simulink model "Sub4"  (R2024a)
settings: Solver=FixedStepDiscrete  StartTime=0.0  StopTime=4.5  FixedStep=75e-6  RelTol=1e-3  EnableMultiTasking=on
undefined symbols (not defined in the file or in its folder): D1, D11, Delta
libraries: spsSeriesRLCBranchLib x41, spsLoadFlowBusLib x29, spsDistributedParametersLineLib x19, spsThreePhaseSeriesRLCLoadLib x15, spsThreePhaseTransformerTwoWindingsLib x13, spsThreePhaseParallelRLCLoadLib x11, spsThreePhaseVIMeasurementLib x11, spsSynchronousMachinepuStandardLib x7, spsExcitationSystemLib x7, spsHydraulicTurbineandGovernorLib x7, spsGenericPowerSystemStabilizerLib x7, spsMultiBandPowerSystemStabilizerLib x7
(part 2 of 5)

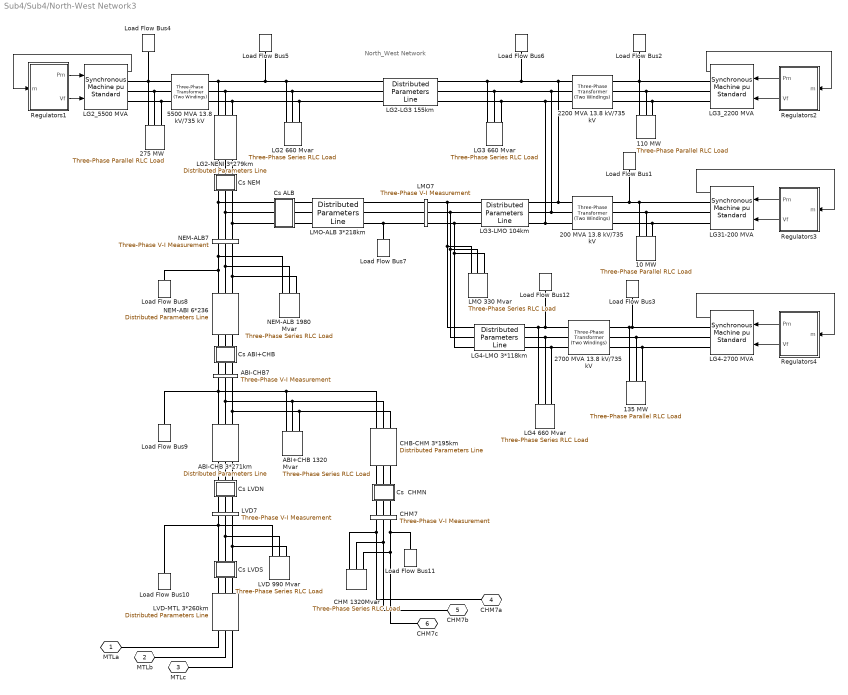
== system Sub4/Sub4/North-West Network3 ==
  note: North_West Network
  10 MW : spsThreePhaseParallelRLCLoadLib/Three-Phase Parallel RLC Load  LConnTagsString=A|B|C  Configuration=Y (grounded)  NominalVoltage=(13800)*1  Vabc=[1e3 1e3 1e3]  Vabcp=[1e3 1e3 1e3]  NominalFrequency=60  UnbalancedPower=off  ActivePower=10000000  InductivePower=0  CapacitivePower=0  Pabc=[10e3 9e3 11e3]  QLabc=[100 90 110]  QCabc=[100 90 110]  Pabcp=[10e3 9e3 11e3]  QLabcp=[100 90 110]  QCabcp=[100 90 110]  Measurements=None  LoadType=constant PQ
  110 MW : spsThreePhaseParallelRLCLoadLib/Three-Phase Parallel RLC Load  LConnTagsString=A|B|C  Configuration=Y (grounded)  NominalVoltage=(13800)*1  Vabc=[1e3 1e3 1e3]  Vabcp=[1e3 1e3 1e3]  NominalFrequency=60  UnbalancedPower=off  ActivePower=110000000  InductivePower=0  CapacitivePower=0  Pabc=[10e3 9e3 11e3]  QLabc=[100 90 110]  QCabc=[100 90 110]  Pabcp=[10e3 9e3 11e3]  QLabcp=[100 90 110]  QCabcp=[100 90 110]  Measurements=None  LoadType=constant PQ
  135 MW : spsThreePhaseParallelRLCLoadLib/Three-Phase Parallel RLC Load  LConnTagsString=A|B|C  Configuration=Y (grounded)  NominalVoltage=(13800)*1  Vabc=[1e3 1e3 1e3]  Vabcp=[1e3 1e3 1e3]  NominalFrequency=60  UnbalancedPower=off  ActivePower=135000000  InductivePower=0  CapacitivePower=0  Pabc=[10e3 9e3 11e3]  QLabc=[100 90 110]  QCabc=[100 90 110]  Pabcp=[10e3 9e3 11e3]  QLabcp=[100 90 110]  QCabcp=[100 90 110]  Measurements=None  LoadType=constant PQ
  200 MVA 13.8 kV/735 kV : spsThreePhaseTransformerTwoWindingsLib/Three-Phase Transformer (Two Windings)  Winding1Connection=Delta (D1)  Winding2Connection=Yg  CoreType=Three single-phase transformers  SetSaturation=off  Hysteresis=off  DataFile='basic_model'  SetInitialFlux=off  Measurements=None  UNITS=pu  NominalPower=[ 200e6 60 ]  Winding1="[ 13.8e3 0.002  0.0]"  Winding2=[ 735e3 0.002 0.12]  Rm=500  Lm=500  L0=0.5  Saturation="[ 0,0  ;  0.005,1.2  ;  1.0,1.4 ]"  InitialFluxes=[ 0.8 , -0.8 , 0.7 ]  BreakLoop=off  DiscreteSolver=Trapezoidal iterative  DataType=off  TransfoNumber=0
  2200 MVA 13.8 kV/735 kV : spsThreePhaseTransformerTwoWindingsLib/Three-Phase Transformer (Two Windings)  Winding1Connection=Delta (D1)  Winding2Connection=Yg  CoreType=Three single-phase transformers  SetSaturation=off  Hysteresis=off  DataFile='basic_model'  SetInitialFlux=off  Measurements=None  UNITS=pu  NominalPower=[ 2200e6 60 ]  Winding1="[ 13.8e3 0.002  0.0]"  Winding2=[ 735e3 0.002 0.12]  Rm=500  Lm=500  L0=0.5  Saturation="[ 0,0  ;  0.005,1.2  ;  1.0,1.4 ]"  InitialFluxes=[ 0.8 , -0.8 , 0.7 ]  BreakLoop=off  DiscreteSolver=Trapezoidal iterative  DataType=off  TransfoNumber=0
  2700 MVA 13.8 kV/735 kV : spsThreePhaseTransformerTwoWindingsLib/Three-Phase Transformer (Two Windings)  Winding1Connection=Delta (D1)  Winding2Connection=Yg  CoreType=Three single-phase transformers  SetSaturation=off  Hysteresis=off  DataFile='basic_model'  SetInitialFlux=off  Measurements=None  UNITS=pu  NominalPower=[ 2700e6 60 ]  Winding1="[ 13.8e3 0.002  0.0]"  Winding2=[ 735e3 0.002 0.12]  Rm=500  Lm=500  L0=0.5  Saturation="[ 0,0  ;  0.005,1.2  ;  1.0,1.4 ]"  InitialFluxes=[ 0.8 , -0.8 , 0.7 ]  BreakLoop=off  DiscreteSolver=Trapezoidal iterative  DataType=off  TransfoNumber=0
  275 MW : spsThreePhaseParallelRLCLoadLib/Three-Phase Parallel RLC Load  LConnTagsString=A|B|C  Configuration=Y (grounded)  NominalVoltage=(13800)*1  Vabc=[1e3 1e3 1e3]  Vabcp=[1e3 1e3 1e3]  NominalFrequency=60  UnbalancedPower=off  ActivePower=275000000  InductivePower=0  CapacitivePower=0  Pabc=[10e3 9e3 11e3]  QLabc=[100 90 110]  QCabc=[100 90 110]  Pabcp=[10e3 9e3 11e3]  QLabcp=[100 90 110]  QCabcp=[100 90 110]  Measurements=None  LoadType=constant PQ
  5500 MVA 13.8 kV/735 kV : spsThreePhaseTransformerTwoWindingsLib/Three-Phase Transformer (Two Windings)  Winding1Connection=Delta (D1)  Winding2Connection=Yg  CoreType=Three single-phase transformers  SetSaturation=off  Hysteresis=off  DataFile='basic_model'  SetInitialFlux=off  Measurements=None  UNITS=pu  NominalPower=[ 5500e6 60 ]  Winding1="[ 13.8e3 0.002  0.0]"  Winding2=[ 735e3 0.002 0.12]  Rm=500  Lm=500  L0=0.5  Saturation="[ 0,0  ;  0.005,1.2  ;  1.0,1.4 ]"  InitialFluxes=[ 0.8 , -0.8 , 0.7 ]  BreakLoop=off  DiscreteSolver=Trapezoidal iterative  DataType=off  TransfoNumber=0
  ABI+CHB 1320 Mvar : spsThreePhaseSeriesRLCLoadLib/Three-Phase Series RLC Load  LConnTagsString=A|B|C  Configuration=Y (grounded)  NominalVoltage=735e3  Vabc=[1e3 1e3 1e3]  Vabcp=[1e3 1e3 1e3]  NominalFrequency=60  UnbalancedPower=off  ActivePower=4400000  InductivePower=1320e6  CapacitivePower=0  Pabc=[10e3 9e3 11e3]  QLabc=[100 90 110]  QCabc=[100 90 110]  Pabcp=[10e3 9e3 11e3]  QLabcp=[100 90 110]  QCabcp=[100 90 110]  Measurements=None  LoadType=constant Z
  ABI-CHB 3*271km : spsDistributedParametersLineLib/Distributed Parameters Line  Phases=3  Length=271  Frequency=60  Resistance="[0.01273  0.3864]/3"  Inductance="[0.9337e-3  4.1264e-3]/3"  Capacitance=[12.74e-9 7.751e-9]*3  x1=[-0.001575 2.80962252870906e-08 -103484.456536303 -819305.847115616;-0.0015 2.82171345098539e-08 -80280.8596539916 -821903.919579672;-0.001425 2.83154873870267e-08 -57013.0874808114 -823844.974625968;-0.00135 2.83912052968237e-08 -33699.7399178284 -825127.4606048;-0.001275 2.84442277115065e-08 -10359.4532983786 -825750.352316497;-0.0012 2.8474512245768e-08 12989.1145095332 -825713.151830956;-0.001125 2.84820346906148e-08 36327.2990180461 -825015.888885677;-0.00105 2.84667890327198e-08 59636.4440395503 -823659.120861989;-0.000975 2.84287874592284e-08 82897.9166001574 -821643.93233949;-0.0009 2.83680603480172e-08 106093.121834615 -818971.934229054;-0.000825 2.82846562434096e-08 129203.517850757 -815645.262485085;-0.00075 2.81786418173708e-08 152210.63055161 -811666.576398077;-0.000675 2.80501018162109e-08 175096.0684033 -807039.056468812;-0.0006 2.78991389928401e-08 197841.537136968 -801766.401865916;-0.000525 2.77258740246295e-08 220428.854372927 -795852.827468807;-0.00045 2.75304454169437e-08 242839.964155374 -789303.060498376;-0.000375 2.73130093924216e-08 265056.951386051 -782122.336738124;-0.0003 2.70737397660942e-08 287062.056145297 -774316.396348756;-0.000225 2.68128278064399e-08 308837.687889058 -765891.479279586;-0.00015 2.65304820824872e-08 330366.439510495 -756854.320280412;-7.5e-05 2.62269282970877e-08 351631.101254964 -747212.143517865]  x2=[-0.001575 6.39240813487654e-08 -329701.15801167 -748762.187115756;-0.0015 6.41301801382965e-08 -308401.441010082 -757783.743021244;-0.001425 6.42850142430497e-08 -286855.19261525 -766199.538197041;-0.00135 6.43884598910107e-08 -265079.636568473 -774002.845185249;-0.001275 6.44404343893114e-08 -243092.179916078 -781187.426141657;-0.0012 6.44408961903329e-08 -220910.399094493 -787747.537822176;-0.001125 6.43898449249186e-08 -198552.025879915 -793677.936173901;-0.00105 6.4287321402669e-08 -176034.933213796 -798973.880527129;-0.000975 6.41334075793192e-08 -153377.12091549 -803631.137384973;-0.0009 6.39282264912245e-08 -130596.701293474 -807645.98380756;-0.000825 6.36719421570073e-08 -107711.88466664 -811015.21038809;-0.00075 6.33647594464432e-08 -84740.9648072501 -813736.123818384;-0.000675 6.3006923916691e-08 -61702.3043171739 -815806.549041878;-0.0006 6.2598721615998e-08 -38614.3199491035 -817224.830992327;-0.000525 6.21404788550378e-08 -15495.4678844847 -817989.83591684;-0.00045 6.1632561946062e-08 7635.77102007237 -818100.952282185;-0.000375 6.10753769100764e-08 30760.9060061072 -817558.09126364;-0.0003 6.04693691522735e-08 53861.4511945383 -816361.686815997;-0.000225 5.98150231059826e-08 76918.9403629924 -814512.695326666;-0.00015 5.91128618454214e-08 99914.9417074196 -812012.594851153;-7.5e-05 5.8363446667558e-08 122831.072576196 -808863.383931525]  x3=[-0.001575 1.30051771042059e-10 -747.841433918899 -1501.46113433961;-0.0015 1.38144212565734e-10 -705.095036949488 -1522.00231179776;-0.001425 1.46126223719561e-10 -661.784997795856 -1541.32682389527;-0.00135 1.53991423805954e-10 -617.945937840636 -1559.41922291284;-0.001275 1.61733525504303e-10 -573.612901357596 -1576.26504606354;-0.0012 1.69346339896971e-10 -528.821327497782 -1591.85082705408;-0.001125 1.7682378141661e-10 -483.607021960005 -1606.1641068496;-0.00105 1.8415987271088e-10 -438.006128368308 -1619.19344363325;-0.000975 1.91348749420646e-10 -392.055099379312 -1630.92842195254;-0.0009 1.98384664867858e-10 -345.790667542516 -1641.35966104537;-0.000825 2.05261994649362e-10 -299.249815936862 -1650.4788223388;-0.00075 2.11975241132958e-10 -252.469748607023 -1658.27861611483;-0.000675 2.18519037852121e-10 -205.487860823064 -1664.75280733764;-0.0006 2.24888153795879e-10 -158.341709187234 -1669.89622063785;-0.000525 2.31077497590397e-10 -111.068981611788 -1673.70474444954;-0.00045 2.37082121568946e-10 -63.7074671918543 -1676.17533429707;-0.000375 2.4289722572699e-10 -16.2950259974044 -1677.3060152287;-0.0003 2.4851816155924e-10 31.1304411915056 -1677.0958833954;-0.000225 2.53940435775595e-10 78.5310231820388 -1675.54510677334;-0.00015 2.5915971389301e-10 125.868828674205 -1672.65492502962;-7.5e-05 2.64171823700416e-10 173.106016550587 -1668.42764853132]  x4=[-0.001575 1.94160017785796e-10 -7080.29438162629 -14859.1258761648;-0.0015 1.90056959794632e-10 -6657.38891400296 -15053.3510061753;-0.001425 1.85801973177776e-10 -6229.16163154324 -15235.5427177154;-0.00135 1.81398459306428e-10 -5795.95485258464 -15405.5553695186;-0.001275 1.768499382822e-10 -5358.11487599796 -15563.2530560724;-0.0012 1.72160046123204e-10 -4915.99170436132 -15708.5097162588;-0.001125 1.67332531857473e-10 -4469.9387641734 -15841.2092341263;-0.00105 1.6237125452605e-10 -4020.31262332977 -15961.2455317107;-0.000975 1.57280180098122e-10 -3567.47270608789 -16068.5226538323;-0.0009 1.52063378300691e-10 -3111.78100574892 -16162.9548448011;-0.000825 1.46725019365294e-10 -2653.60179528581 -16244.4666169684;-0.00075 1.41269370694385e-10 -2193.30133614901 -16312.9928110708;-0.000675 1.35700793450036e-10 -1731.24758548273 -16368.4786483172;-0.0006 1.30023739067695e-10 -1267.80990198559 -16410.8797741782;-0.000525 1.24242745697774e-10 -803.35875065095 -16440.1622938426;-0.00045 1.18362434577919e-10 -338.265406622837 -16456.3027993123;-0.000375 1.12387506338869e-10 127.098341595695 -16459.2883881141;-0.0003 1.06322737246837e-10 592.360489344626 -16449.1166736139;-0.000225 1.00172975385444e-10 1057.14911318179 -16425.7957869249;-0.00015 9.39431367802247e-11 1521.09266819281 -16389.3443704068;-7.5e-05 8.76382014688418e-11 1983.82028499837 -16339.7915627644]  x5=0.00153261764655846  V1=ones(3,3)  V2=ones(3,3)  I1=ones(3,3)  I2=ones(3,3)  nHarmo=1  Measurements=None  Decoupling=on  VsMag0=[674275.598206343 674275.04688363 674275.387112461]  VrMag0=[668005.988427244 668005.867389034 668005.726368297]  VsAngle0=[-3.17875639507245 -123.178750059774 116.821287344148]  VrAngle0=[-19.7452308032692 -139.745250763834 100.254768207195]  IsMag0=[1378.35069563154 1378.34088888526 1378.33344706121]  IrMag0=[13525.2461163755 13525.2482026067 13525.2572474119]  IsAngle0=[-22.4561903612897 -142.456782921022 97.5438663998778]  IrAngle0=[-21.4575985540855 -141.457549208479 98.5424184650439]
      settings: AttributesFormatString=\n  LibrarySourceBlock=sps_lib/Power Grid Elements/Distributed Parameters Line
  ABI-CHB7 : spsThreePhaseVIMeasurementLib/Three-Phase V-I Measurement  VoltageMeasurement=no  SetLabelV=on  LabelV=Vabc_ABI7  Vpu=on  VpuLL=off  CurrentMeasurement=no  SetLabelI=off  LabelI=A1  Ipu=off  Pbase=100e6  Vbase=500e3  OutputType=Magnitude  PhasorSimulation=off  PSBequivalent=0
  CHB-CHM 3*195km : spsDistributedParametersLineLib/Distributed Parameters Line  Phases=3  Length=195  Frequency=60  Resistance="[0.01273  0.3864]/3"  Inductance="[0.9337e-3  4.1264e-3]/3"  Capacitance=[12.74e-9 7.751e-9]*3  x1=[-0.001125 2.84820346906148e-08 0 0;-0.00105 2.84667890327198e-08 0 0;-0.000975 2.84287874592284e-08 0 0;-0.0009 2.83680603480172e-08 0 0;-0.000825 2.82846562434096e-08 0 0;-0.00075 2.81786418173708e-08 0 0;-0.000675 2.80501018162109e-08 175096.0684033 -807039.056468812;-0.0006 2.78991389928401e-08 197841.537136968 -801766.401865916;-0.000525 2.77258740246295e-08 220428.854372927 -795852.827468807;-0.00045 2.75304454169437e-08 242839.964155374 -789303.060498376;-0.000375 2.73130093924216e-08 265056.951386051 -782122.336738124;-0.0003 2.70737397660942e-08 287062.056145297 -774316.396348756;-0.000225 2.68128278064399e-08 308837.687889058 -765891.479279586;-0.00015 2.65304820824872e-08 330366.439510495 -756854.320280412;-7.5e-05 2.62269282970877e-08 351631.101254964 -747212.143517865]  x2=[-0.001125 1.9148732573154e-08 0 0;-0.00105 1.90857883031073e-08 0 0;-0.000975 1.90075871459134e-08 0 0;-0.0009 1.8914191614381e-08 0 0;-0.000825 1.88056763674688e-08 0 0;-0.00075 1.8682128150605e-08 0 0;-0.000675 1.85436457263437e-08 86661.6913680095 -814290.34412733;-0.0006 1.83903397954161e-08 109647.510746575 -811514.902082727;-0.000525 1.82223329082377e-08 132545.679582712 -808090.747441994;-0.00045 1.80397593669435e-08 155337.893430608 -804020.617421958;-0.000375 1.78427651180289e-08 178005.932543245 -799307.765622284;-0.0003 1.76315076356824e-08 200531.676436989 -793955.95942459;-0.000225 1.7406155795903e-08 222897.118376827 -787969.476980865;-0.00015 1.71668897415036e-08 245084.379770675 -781353.103793579;-7.5e-05 1.6913900738107e-08 267075.72446125 -774112.128890224]  x3=[-0.001125 1.05074727479882e-10 0 0;-0.00105 1.03081983403571e-10 0 0;-0.000975 1.01006837166934e-10 0 0;-0.0009 9.88509476101221e-11 0 0;-0.000825 9.66160381182611e-11 0 0;-0.00075 9.43038952438033e-11 0 0;-0.000675 9.19163672783856e-11 335.259499975439 -5255.16303225201;-0.0006 8.94553627753332e-11 483.692851575089 -5243.58412650876;-0.000525 8.69228490239911e-11 631.739546509938 -5227.81357984431;-0.00045 8.43208504771034e-11 779.281238517247 -5207.86399899236;-0.000375 8.16514471324966e-11 926.199985025888 -5183.7513313426;-0.0003 7.89167728703611e-11 1072.37834143783 -5155.49485219263;-0.000225 7.61190137474601e-11 1217.69945501157 -5123.11714933953;-0.00015 7.32604062496294e-11 1362.0471582724 -5086.64410502357;-7.5e-05 7.03432355039646e-11 1505.30606187493 -5046.10487523832]  x4=[-0.001125 7.89655264948449e-11 0 0;-0.00105 8.1703463998163e-11 0 0;-0.000975 8.4376089002466e-11 0 0;-0.0009 8.69812650522178e-11 0 0;-0.000825 8.95169096095449e-11 0 0;-0.00075 9.19809957189847e-11 0 0;-0.000675 9.43715536278032e-11 265.942029612222 -12956.0177279497;-0.0006 9.66866723605848e-11 632.108856779635 -12943.3211843352;-0.000525 9.89245012468371e-11 997.770385798528 -12920.2779478054;-0.00045 1.01083251400388e-10 1362.63431243741 -12886.906438771;-0.000375 1.03161197149396e-10 1726.40897005594 -12843.2333339057;-0.0003 1.05156677415821e-10 2088.80356275875 -12789.2935448214;-0.000225 1.07068097043271e-10 2449.52839785325 -12725.1301901601;-0.00015 1.08893928072142e-10 2808.29511742555 -12650.7945611258;-7.5e-05 1.10632710961045e-10 3164.81692884934 -12566.346080483]  x5=0.0011028060556417  V1=ones(3,3)  V2=ones(3,3)  I1=ones(3,3)  I2=ones(3,3)  nHarmo=1  Measurements=None  Decoupling=on  VsMag0=[674275.598206343 674275.04688363 674275.387112461]  VrMag0=[668620.174918635 668620.122023065 668619.982355123]  VsAngle0=[-3.17875639507245 -123.178750059774 116.821287344148]  VrAngle0=[-9.34509688682596 -129.345113323857 110.654898820144]  IsMag0=[4319.32992808263 4319.31639781902 4319.30396194708]  IrMag0=[10629.3727910758 10629.3784873059 10629.3938662895]  IsAngle0=[-11.7695166369437 -131.7698107405 108.230491745414]  IrAngle0=[-14.2441447349356 -134.24403128562 105.755885398883]
      settings: AttributesFormatString=\n  LibrarySourceBlock=sps_lib/Power Grid Elements/Distributed Parameters Line
  CHM 1320Mvar : spsThreePhaseSeriesRLCLoadLib/Three-Phase Series RLC Load  LConnTagsString=A|B|C  Configuration=Y (grounded)  NominalVoltage=735e3  Vabc=[1e3 1e3 1e3]  Vabcp=[1e3 1e3 1e3]  NominalFrequency=60  UnbalancedPower=off  ActivePower=4400000  InductivePower=1320e6  CapacitivePower=0  Pabc=[10e3 9e3 11e3]  QLabc=[100 90 110]  QCabc=[100 90 110]  Pabcp=[10e3 9e3 11e3]  QLabcp=[100 90 110]  QCabcp=[100 90 110]  Measurements=None  LoadType=constant Z
  CHM7 : spsThreePhaseVIMeasurementLib/Three-Phase V-I Measurement  VoltageMeasurement=no  SetLabelV=on  LabelV=Vabc_CHM7  Vpu=on  VpuLL=off  CurrentMeasurement=no  SetLabelI=off  LabelI=A1  Ipu=off  Pbase=100e6  Vbase=735e3  OutputType=Magnitude  PhasorSimulation=off  PSBequivalent=0
  "Cs  CHMN " : Subsystem  mask{Xc=25/3}
      mask prompts: Xc "Condensator Reactance at  60Hz  (ohm):"
      mask help: Series Compensation
      mask init:
      | Cs=1/Xc/(2*pi*60);
      mask Display: disp('Cs')
  "Cs ABI+CHB " : Subsystem  mask{Xc=25/6}
      mask prompts: Xc "Condensator Reactance at  60Hz  (ohm):"
      mask help: Series Compensation
      mask init:
      | Cs=1/Xc/(2*pi*60);
      mask Display: disp('Cs')
  Cs ALB : Subsystem  mask{Xc=16/3}
      mask prompts: Xc "Reactance @ 60Hz du condensateur (ohm):"
      mask init:
      | Cs=1/Xc/(2*pi*60);
      mask Display: disp('Cs')
  "Cs LVDN " : Subsystem  mask{Xc=34/3}
      mask prompts: Xc "Condensator Reactance at  60Hz  (ohm):"
      mask help: Series Compensation
      mask init:
      | Cs=1/Xc/(2*pi*60);
      mask Display: disp('Cs')
  "Cs LVDS " : Subsystem  mask{Xc=34/3}
      mask prompts: Xc "Condensator Reactance at  60Hz  (ohm):"
      mask help: Series Compensation
      mask init:
      | Cs=1/Xc/(2*pi*60);
      mask Display: disp('Cs')
  "Cs NEM " : Subsystem  mask{Xc=16/3}
      mask prompts: Xc "Condensator Reactance at  60Hz  (ohm):"
      mask help: Series Compensation
      mask init:
      | Cs=1/Xc/(2*pi*60);
      mask Display: disp('Cs')
  LG2 660 Mvar : spsThreePhaseSeriesRLCLoadLib/Three-Phase Series RLC Load  LConnTagsString=A|B|C  Configuration=Y (grounded)  NominalVoltage=735e3  Vabc=[1e3 1e3 1e3]  Vabcp=[1e3 1e3 1e3]  NominalFrequency=60  UnbalancedPower=off  ActivePower=2200000  InductivePower=660e6  CapacitivePower=0  Pabc=[10e3 9e3 11e3]  QLabc=[100 90 110]  QCabc=[100 90 110]  Pabcp=[10e3 9e3 11e3]  QLabcp=[100 90 110]  QCabcp=[100 90 110]  Measurements=None  LoadType=constant Z
  LG2-LG3 155km : spsDistributedParametersLineLib/Distributed Parameters Line  Phases=3  Length=155  Frequency=60  Resistance="[0.01273  0.3864]"  Inductance="[0.9337e-3  4.1264e-3]"  Capacitance=[12.74e-9 7.751e-9]  x1=[-0.0009 5.06919408838322e-10 371984.249881669 -674633.962928252;-0.000825 5.50165803284005e-10 390907.835511608 -663848.049238563;-0.00075 5.92972403604362e-10 409518.935398929 -652531.465575529;-0.000675 6.35304990858059e-10 427802.672115142 -640693.258242979;-0.0006 6.77129725022557e-10 445744.429920867 -628342.890522726;-0.000525 7.18413172045304e-10 463329.866449431 -615490.235109758;-0.00045 7.59122330570408e-10 480544.92417194 -602145.566220159;-0.000375 7.99224658319416e-10 497375.84163465 -588319.55137806;-0.0003 8.3868809810511e-10 513809.164459663 -574023.24288818;-0.000225 8.77481103457537e-10 529831.756100151 -559268.069000786;-0.00015 9.15572663841771e-10 545430.80834151 -544065.82477612;-7.5e-05 9.52932329447262e-10 560593.851540052 -528428.662655615]  x2=[-0.0009 -2.17943716120966e-10 375373.731714279 -666225.896356748;-0.000825 -2.67147501271516e-10 394058.262242218 -655347.523813034;-0.00075 -3.16137732797043e-10 412427.788624615 -643945.276485937;-0.000675 -3.64875248656041e-10 430467.626543143 -632028.269157511;-0.0006 -4.13321088824043e-10 448163.355227387 -619606.028101077;-0.000525 -4.61436526437663e-10 465500.828982591 -606688.483466069;-0.00045 -5.09183098752265e-10 482466.188497509 -593285.961340023;-0.000375 -5.56522637888486e-10 499045.871923322 -579409.175494062;-0.0003 -6.03417301343062e-10 515226.625714777 -565069.218818469;-0.000225 -6.49829602239538e-10 530995.515224868 -550277.5544552;-0.00015 -6.9572243929471e-10 546339.935044591 -535046.00663443;-7.5e-05 -7.4105912647682e-10 561247.619079521 -519386.751222434]  x3=[-0.0009 1.00594082995822e-11 1272.11889165525 -2673.50704029727;-0.000825 9.91695925489918e-12 1347.19195646224 -2636.47471081232;-0.00075 9.76658274472235e-12 1421.18809663195 -2597.33482378297;-0.000675 9.60839897773311e-12 1494.04816078213 -2556.11866703604;-0.0006 9.44253440361452e-12 1565.71390569229 -2512.8591881366;-0.000525 9.26912161196929e-12 1636.12804286246 -2467.59096805021;-0.00045 9.08829922632977e-12 1705.23428430876 -2420.35019349936;-0.000375 8.90021179334436e-12 1772.97738755914 -2371.17462803643;-0.0003 8.70500966722916e-12 1839.30319981338 -2320.10358185604;-0.000225 8.50284888957709e-12 1904.15870123196 -2267.17788037108;-0.00015 8.29389106462065e-12 1967.49204731939 -2212.43983157754;-7.5e-05 8.07830323004793e-12 2029.25261036783 -2155.93319223411]  x4=[-0.0009 -1.23049206033618e-11 974.452643997113 -2530.47846704131;-0.000825 -1.21578095802014e-11 1045.60107405548 -2501.91852232224;-0.00075 -1.20009797900833e-11 1115.91366661349 -2471.35858221706;-0.000675 -1.18345566003422e-11 1185.33421486045 -2438.82307587431;-0.0006 -1.16586730471295e-11 1253.80722507228 -2404.33801167996;-0.000525 -1.14734697290666e-11 1321.27796097228 -2367.93095646667;-0.00045 -1.12790946948523e-11 1387.6924874865 -2329.63101347734;-0.000375 -1.10757033249148e-11 1452.99771385864 -2289.46879910038;-0.0003 -1.08634582072034e-11 1517.14143608993 -2247.47641839548;-0.000225 -1.06425290072176e-11 1580.07237867025 -2203.68743942925;-0.00015 -1.04130923323796e-11 1641.74023556698 -2158.13686644149;-7.5e-05 -1.01753315908567e-11 1702.09571043887 -2110.86111186329]  x5=0.000876589428843401  V1=ones(3,3)  V2=ones(3,3)  I1=ones(3,3)  I2=ones(3,3)  nHarmo=1  Measurements=None  Decoupling=on  VsMag0=[629022.539261933 629021.416248083 629022.998971787]  VrMag0=[624373.329666387 624372.279031931 624373.793133007]  VsAngle0=[18.3117620160156 -101.688130574181 138.311904308248]  VrAngle0=[18.8383509464065 -101.161544280635 138.838486827798]  IsMag0=[2426.25467785361 2426.24994282972 2426.25518358313]  IrMag0=[2222.1103547092 2222.10693756296 2222.11326012537]  IsAngle0=[14.8862320606511 -105.113689591384 134.886368071068]  IrAngle0=[10.501009655439 -109.498852970967 130.501154646769]
      settings: AttributesFormatString=\n  LibrarySourceBlock=sps_lib/Power Grid Elements/Distributed Parameters Line
  LG2-NENI 3*279km : spsDistributedParametersLineLib/Distributed Parameters Line  Phases=3  Length=279  Frequency=60  Resistance="[0.01273  0.3864]/3"  Inductance="[0.9337e-3  4.1264e-3]/3"  Capacitance=[12.74e-9 7.751e-9]*3  x1=[-0.00165 5.80103510672884e-11 168997.444323772 -751627.644710306;-0.001575 1.03709164490765e-10 190178.800706824 -746549.517209881;-0.0015 1.49325074394951e-10 211208.131066425 -740874.60944799;-0.001425 1.94821616119417e-10 232068.624877643 -734607.457859067;-0.00135 2.40162420424827e-10 252743.606580903 -727753.072308203;-0.001275 2.85311242565958e-10 273216.54891217 -720316.932086331;-0.0012 3.3023199126519e-10 293471.086114589 -712304.981530168;-0.001125 3.74888757563323e-10 313491.027021026 -703723.625270402;-0.00105 4.19245843524651e-10 333260.367997037 -694579.723111926;-0.000975 4.63267790773341e-10 352763.305733925 -684880.584550222;-0.0009 5.06919408838322e-10 371984.249881669 -674633.962928252;-0.000825 5.50165803284005e-10 390907.835511608 -663848.049238563;-0.00075 5.92972403604362e-10 409518.935398929 -652531.465575529;-0.000675 6.3530499085806e-10 427802.672115142 -640693.258242979;-0.0006 6.77129725022557e-10 445744.429920867 -628342.890522726;-0.000525 7.18413172045304e-10 463329.866449431 -615490.235109758;-0.00045 7.59122330570408e-10 480544.92417194 -602145.566220159;-0.000375 7.99224658319416e-10 497375.84163465 -588319.55137806;-0.0003 8.3868809810511e-10 513809.164459663 -574023.24288818;-0.000225 8.77481103457537e-10 529831.756100151 -559268.069000786;-0.00015 9.15572663841771e-10 545430.80834151 -544065.82477612;-7.5e-05 9.52932329447262e-10 560593.851540052 -528428.662655615]  x2=[-0.00165 1.6193520704975e-08 -47534.3064648496 -809002.983106388;-0.001575 1.62743303650456e-08 -24644.3461226266 -810023.426229919;-0.0015 1.63421305744279e-08 -1734.68546718411 -810396.349020296;-0.001425 1.63968671346721e-08 21176.3618692791 -810121.453368747;-0.00135 1.64384962902092e-08 44070.4811460734 -809198.959022648;-0.001275 1.64669847633294e-08 66929.3711545403 -807629.603409866;-0.0012 1.64823097807832e-08 89734.7588477601 -805414.641049265;-0.001125 1.64844590919859e-08 112468.413947745 -802555.842547867;-0.00105 1.64734309788112e-08 135112.163518444 -799055.493185452;-0.000975 1.6449234256964e-08 157647.906492912 -794916.391087744;-0.0009 1.64118882689335e-08 180057.628143024 -790141.844989629;-0.000825 1.63614228685311e-08 202323.414480172 -784735.671590205;-0.00075 1.62978783970258e-08 224427.466575436 -778702.19250177;-0.000675 1.62213056508958e-08 246352.114787776 -772046.230795192;-0.0006 1.61317658412228e-08 268079.832888868 -764773.10714442;-0.000525 1.60293305447605e-08 289593.252073308 -756888.635573217;-0.00045 1.59140816467178e-08 310875.174842966 -748399.118807522;-0.000375 1.57861112753004e-08 331908.588754403 -739311.343237143;-0.0003 1.5645521728065e-08 352676.680018363 -729632.573490822;-0.000225 1.54924253901448e-08 373162.846940449 -719370.546629006;-0.00015 1.53269446444097e-08 393350.713192275 -708533.465958953;-7.5e-05 1.5149211773636e-08 413224.140902443 -697129.994477139]  x3=[-0.00165 1.33127872984606e-11 -1677.04894977063 -1941.35400834447;-0.001575 1.64197410331452e-11 -1621.49508617435 -1987.98793711556;-0.0015 1.95135690780784e-11 -1564.64502421588 -2033.03269874696;-0.001425 2.25917982744581e-11 -1506.54420896492 -2076.45228514542;-0.00135 2.56519679329634e-11 -1447.23908532422 -2118.21198735793;-0.001275 2.86916318007913e-11 -1386.7770609022 -2158.27842331746;-0.0012 3.17083600171544e-11 -1325.20646811611 -2196.61956452817;-0.001125 3.46997410556739e-11 -1262.57652555574 -2233.2047616684;-0.00105 3.76633836521174e-11 -1198.93729863891 -2268.00476909133;-0.000975 4.05969187159384e-11 -1134.3396595899 -2300.99176820349;-0.0009 4.34980012240916e-11 -1068.835246773 -2332.1393897025;-0.000825 4.6364312095608e-11 -1002.47642341355 -2361.4227346563;-0.00075 4.9193560045433e-11 -935.316235739635 -2388.81839440701;-0.000675 5.19834834160443e-11 -867.408370577684 -2414.30446928337;-0.0006 5.47318519853868e-11 -798.807112436086 -2437.86058610709;-0.000525 5.74364687496777e-11 -729.567300110966 -2459.46791447878;-0.00045 6.00951716796574e-11 -659.74428284889 -2479.10918183077;-0.000375 6.27058354488835e-11 -589.393876101532 -2496.76868723444;-0.0003 6.52663731326831e-11 -518.572316907646 -2512.43231395138;-0.000225 6.77747378764094e-11 -447.336218938047 -2526.08754071805;-0.00015 7.02289245316657e-11 -375.742527239503 -2537.7234517551;-7.5e-05 7.26269712591898e-11 -303.848472713737 -2547.3307454933]  x4=[-0.00165 4.10856122854733e-11 -141.249463963346 -15427.0315937102;-0.001575 3.88754417479028e-11 294.936850750049 -15424.8591939222;-0.0015 3.66341947770132e-11 730.887397457643 -15410.3563977029;-0.001425 3.43636629913407e-11 1166.25368396266 -15383.5347983656;-0.00135 3.20656614192547e-11 1600.687685117 -15344.4158366864;-0.001275 2.97420270480513e-11 2033.8421210272 -15293.0307837649;-0.0012 2.73946173554938e-11 2465.37073466467 -15229.420716026;-0.001125 2.50253088249741e-11 2894.92856865829 -15153.6364823847;-0.00105 2.26359954454798e-11 3322.17224104802 -15065.7386635978;-0.000975 2.02285871975687e-11 3746.7602197792 -14965.7975238367;-0.0009 1.78050085265597e-11 4168.35309571804 -14853.8929545195;-0.000825 1.53671968041602e-11 4586.6138539701 -14730.1144104466;-0.00075 1.29171007797615e-11 5001.20814328484 -14594.5608382923;-0.000675 1.04566790226378e-11 5411.8045433309 -14447.3405975081;-0.0006 7.98789835629589e-12 5818.07482962839 -14288.571373702;-0.000525 5.51273228622691e-12 6219.69423592662 -14118.3800845623;-0.00045 3.03315942231595e-12 6616.34171381716 -13936.9027784014;-0.000375 5.51161897171696e-13 7007.70018937509 -13744.2845254012;-0.0003 -1.9312762183601e-12 7393.45681662305 -13540.679301646;-0.000225 -4.41217050123246e-12 7773.30322761548 -13326.2498660364;-0.00015 -6.8895377625146e-12 8146.93577894329 -13101.1676301824;-7.5e-05 -9.36139763272286e-12 8514.0557944617 -12865.6125213794]  x5=0.00157786097191812  V1=ones(3,3)  V2=ones(3,3)  I1=ones(3,3)  I2=ones(3,3)  nHarmo=1  Measurements=None  Decoupling=on  VsMag0=[629022.539261933 629021.416248083 629022.998971787]  VrMag0=[661687.482462953 661686.807299191 661687.362395074]  VsAngle0=[18.3117620160156 -101.688130574181 138.311904308248]  VrAngle0=[2.27736225154332 -117.722616000124 122.277423755893]  IsMag0=[2108.44631509133 2108.42876135602 2108.41340422822]  IrMag0=[12679.5195981426 12679.5310413664 12679.5487055218]  IsAngle0=[-35.1815546032586 -155.182311890514 84.8184798659538]  IrAngle0=[5.11533890202494 -114.884539075258 125.115355131992]
      settings: AttributesFormatString=\n  LibrarySourceBlock=sps_lib/Power Grid Elements/Distributed Parameters Line
  LG2_5500 MVA : spsSynchronousMachinepuStandardLib/Synchronous Machine pu Standard  PresetModel=No  MechanicalLoad=Mechanical power Pm  ShowDetailedParameters=on  RotorType=Salient-pole  Units=per unit standard parameters  MeasurementBus=off  NominalParameters="[5500E6  13800   60 ]"  Reactances1=[ 31 32 33 34 35 36 37 ]  Reactances2=[ 1.305, 0.296, 0.252, 0.474, 0.243, 0.18 ]  dAxisTimeConstants=Short-circuit  qAxisTimeConstants=Open-circuit  TimeConstants1=[]  TimeConstants2=[]  TimeConstants3=[]  TimeConstants4=[]  TimeConstants5=[ 1.01, 0.053, 0.1 ]  TimeConstants6=[]  TimeConstants7=[]  TimeConstants8=[]  StatorResistance=2.8544e-3  Mechanical="[ 4.1  0  32]"  PolePairs=32  InitialConditions=[0 -65.2434 0.985682 0.985682 0.985682 -1.22427 -121.224 118.776 1.47412]  SetSaturation=off  Saturation=[0.6404,0.7127,0.8441,0.9214,0.9956,1.082,1.19,1.316,1.457;0.7,0.7698,0.8872,0.9466,0.9969,1.046,1.1,1.151,1.201]  LoadFlowParameters=[2 4000000000 0 0 0]  TsPowergui=0  TsBlock=-1  IterativeModel=Trapezoidal non iterative  IterativeDiscreteModel=Trapezoidal non iterative  BusType=swing  Pref=0  Qref=0  Qmin=-Inf  Qmax=Inf  PLF=0  QLF=0
  LG3 660 Mvar : spsThreePhaseSeriesRLCLoadLib/Three-Phase Series RLC Load  LConnTagsString=A|B|C  Configuration=Y (grounded)  NominalVoltage=735e3  Vabc=[1e3 1e3 1e3]  Vabcp=[1e3 1e3 1e3]  NominalFrequency=60  UnbalancedPower=off  ActivePower=2200000  InductivePower=660e6  CapacitivePower=0  Pabc=[10e3 9e3 11e3]  QLabc=[100 90 110]  QCabc=[100 90 110]  Pabcp=[10e3 9e3 11e3]  QLabcp=[100 90 110]  QCabcp=[100 90 110]  Measurements=None  LoadType=constant Z
  LG3-LMO 104km : spsDistributedParametersLineLib/Distributed Parameters Line  Phases=3  Length=104  Frequency=60  Resistance="[0.01273  0.3864]"  Inductance="[0.9337e-3  4.1264e-3]"  Capacitance=[12.74e-9 7.751e-9]  x1=[-0.0006 -4.13321088824043e-10 0 0;-0.000525 -4.61436526437663e-10 0 0;-0.00045 -5.09183098752265e-10 0 0;-0.000375 -5.56522637888486e-10 499045.871923322 -579409.175494062;-0.0003 -6.03417301343062e-10 515226.625714777 -565069.218818469;-0.000225 -6.49829602239538e-10 530995.515224868 -550277.5544552;-0.00015 -6.9572243929471e-10 546339.935044591 -535046.00663443;-7.5e-05 -7.4105912647682e-10 561247.619079521 -519386.751222434]  x2=[-0.0006 4.66666036101226e-09 0 0;-0.000525 4.59046460778431e-09 0 0;-0.00045 4.51059930738535e-09 0 0;-0.000375 4.42712830291456e-09 445735.71370671 -651849.764162774;-0.0003 4.34011831981575e-09 463985.717973658 -638987.984734865;-0.000225 4.24963891253812e-09 481864.819156877 -625615.408088803;-0.00015 4.15576240893545e-09 499358.724976442 -611742.724057751;-7.5e-05 4.05856385244839e-09 516453.451071705 -597381.022253065]  x3=[-0.0006 1.11305091875994e-11 0 0;-0.000525 1.18778571843415e-11 0 0;-0.00045 1.26157102037879e-11 0 0;-0.000375 1.33434784175241e-11 -337.815764584762 -872.913223711573;-0.0003 1.40605800587755e-11 -313.002403558919 -882.114195189639;-0.000225 1.4766441887462e-11 -287.938833200769 -890.61001807687;-0.00015 1.54604996484377e-11 -262.645088944969 -898.39390094244;-7.5e-05 1.61421985225481e-11 -237.141390223672 -905.459621469485]  x4=[-0.0006 -6.69849071160608e-12 0 0;-0.000525 -7.49016271277685e-12 0 0;-0.00045 -8.27584719247836e-12 0 0;-0.000375 -9.05491608655891e-12 3507.69484614572 -3894.26054707419;-0.0003 -9.82674661926473e-12 3616.38515846558 -3793.5395268898;-0.000225 -1.05907218010774e-11 3722.1845878223 -3689.7860092507;-0.00015 -1.13462309219257e-11 3825.00855977085 -3583.08293313143;-7.5e-05 -1.20926700393782e-11 3924.77487840132 -3473.51559533843]  x5=0.000588163229675572  V1=ones(3,3)  V2=ones(3,3)  I1=ones(3,3)  I2=ones(3,3)  nHarmo=1  Measurements=None  Decoupling=on  VsMag0=[624373.329666387 624372.279031931 624373.793133007]  VrMag0=[644768.423999943 644767.634896107 644768.519320875]  VsAngle0=[18.8383509464065 -101.161544280635 138.838486827798]  VrAngle0=[12.4643674245489 -107.535582309766 132.464453284623]  IsMag0=[766.124869864333 766.121415585298 766.108315941495]  IrMag0=[4289.80561922853 4289.81652389758 4289.82131843397]  IsAngle0=[-43.0551695781835 -163.05644995892 76.9444139609737]  IrAngle0=[20.1104998668519 -99.8893421012226 140.110452750547]
      settings: AttributesFormatString=\n  LibrarySourceBlock=sps_lib/Power Grid Elements/Distributed Parameters Line
  LG31-200 MVA : spsSynchronousMachinepuStandardLib/Synchronous Machine pu Standard  PresetModel=No  MechanicalLoad=Mechanical power Pm  ShowDetailedParameters=on  RotorType=Salient-pole  Units=per unit standard parameters  MeasurementBus=off  NominalParameters="[200E6  13800   60 ]"  Reactances1=[ 31 32 33 34 35 36 37 ]  Reactances2=[ 1.305, 0.296, 0.252, 0.474, 0.243, 0.18 ]  dAxisTimeConstants=Short-circuit  qAxisTimeConstants=Open-circuit  TimeConstants1=[]  TimeConstants2=[]  TimeConstants3=[]  TimeConstants4=[]  TimeConstants5=[ 1.01, 0.053, 0.1 ]  TimeConstants6=[]  TimeConstants7=[]  TimeConstants8=[]  StatorResistance=2.8544e-3  Mechanical="[ 3.2  0  32]"  PolePairs=32  InitialConditions=[0 -67.6291 0.902477 0.902477 0.902477 -4.2812 -124.281 115.719 1.45511]  SetSaturation=off  Saturation=[0.6404,0.7127,0.8441,0.9214,0.9956,1.082,1.19,1.316,1.457;0.7,0.7698,0.8872,0.9466,0.9969,1.046,1.1,1.151,1.201]  LoadFlowParameters=[1 180000000 0 0 0]  TsPowergui=0  TsBlock=-1  IterativeModel=Trapezoidal non iterative  IterativeDiscreteModel=Trapezoidal non iterative  BusType=PV  Pref=180000000  Qref=0  Qmin=-Inf  Qmax=Inf  PLF=0  QLF=0
  LG3_2200 MVA : spsSynchronousMachinepuStandardLib/Synchronous Machine pu Standard  PresetModel=No  MechanicalLoad=Mechanical power Pm  ShowDetailedParameters=on  RotorType=Salient-pole  Units=per unit standard parameters  MeasurementBus=off  NominalParameters="[2200E6  13800   60 ]"  Reactances1=[ 31 32 33 34 35 36 37 ]  Reactances2=[ 1.305, 0.296, 0.252, 0.474, 0.243, 0.18 ]  dAxisTimeConstants=Short-circuit  qAxisTimeConstants=Open-circuit  TimeConstants1=[]  TimeConstants2=[]  TimeConstants3=[]  TimeConstants4=[]  TimeConstants5=[ 1.01, 0.053, 0.1 ]  TimeConstants6=[]  TimeConstants7=[]  TimeConstants8=[]  StatorResistance=2.8544e-3  Mechanical="[ 3.2  0  32]"  PolePairs=32  InitialConditions=[0 -70.0065 0.820496 0.820496 0.820496 -4.90643 -124.906 115.094 1.38903]  SetSaturation=off  Saturation=[0.6404,0.7127,0.8441,0.9214,0.9956,1.082,1.19,1.316,1.457;0.7,0.7698,0.8872,0.9466,0.9969,1.046,1.1,1.151,1.201]  LoadFlowParameters=[1 1800000000 0 0 0]  TsPowergui=0  TsBlock=-1  IterativeModel=Trapezoidal non iterative  IterativeDiscreteModel=Trapezoidal non iterative  BusType=PV  Pref=1800000000  Qref=0  Qmin=-Inf  Qmax=Inf  PLF=0  QLF=0
  LG4 660 Mvar : spsThreePhaseSeriesRLCLoadLib/Three-Phase Series RLC Load  LConnTagsString=A|B|C  Configuration=Y (grounded)  NominalVoltage=735e3  Vabc=[1e3 1e3 1e3]  Vabcp=[1e3 1e3 1e3]  NominalFrequency=60  UnbalancedPower=off  ActivePower=2200000  InductivePower=660e6  CapacitivePower=0  Pabc=[10e3 9e3 11e3]  QLabc=[100 90 110]  QCabc=[100 90 110]  Pabcp=[10e3 9e3 11e3]  QLabcp=[100 90 110]  QCabcp=[100 90 110]  Measurements=None  LoadType=constant Z
  LG4-2700 MVA : spsSynchronousMachinepuStandardLib/Synchronous Machine pu Standard  PresetModel=No  MechanicalLoad=Mechanical power Pm  ShowDetailedParameters=on  RotorType=Salient-pole  Units=per unit standard parameters  MeasurementBus=off  NominalParameters="[2700E6  13800   60 ]"  Reactances1=[ 31 32 33 34 35 36 37 ]  Reactances2=[ 1.305, 0.296, 0.252, 0.474, 0.243, 0.18 ]  dAxisTimeConstants=Short-circuit  qAxisTimeConstants=Open-circuit  TimeConstants1=[]  TimeConstants2=[]  TimeConstants3=[]  TimeConstants4=[]  TimeConstants5=[ 1.01, 0.053, 0.1 ]  TimeConstants6=[]  TimeConstants7=[]  TimeConstants8=[]  StatorResistance=2.8544e-3  Mechanical="[ 3.7  0  32]"  PolePairs=32  InitialConditions=[0 -69.506 0.926038 0.926038 0.926038 -2.40174 -122.402 117.598 1.38766]  SetSaturation=off  Saturation=[0.6404,0.7127,0.8441,0.9214,0.9956,1.082,1.19,1.316,1.457;0.7,0.7698,0.8872,0.9466,0.9969,1.046,1.1,1.151,1.201]  LoadFlowParameters=[1 2500000000 0 0 0]  TsPowergui=0  TsBlock=-1  IterativeModel=Trapezoidal non iterative  IterativeDiscreteModel=Trapezoidal non iterative  BusType=PV  Pref=2500000000  Qref=0  Qmin=-Inf  Qmax=Inf  PLF=0  QLF=0
  LG4-LMO 3*118km : spsDistributedParametersLineLib/Distributed Parameters Line  Phases=3  Length=118  Frequency=60  Resistance="[0.01273  0.3864]/3"  Inductance="[0.9337e-3  4.1264e-3]/3"  Capacitance=[12.74e-9 7.751e-9]*3  x1=[-0.000675 -5.14666934265879e-10 400494.989180222 -665247.597360552;-0.0006 -5.79457249979835e-10 419141.837998085 -653659.450927359;-0.000525 -6.43784356434151e-10 437453.631243737 -641548.77913042;-0.00045 -7.07596831524165e-10 455415.730749838 -628925.263055469;-0.000375 -7.70843664533653e-10 473013.777888872 -615798.993748111;-0.0003 -8.33474296912016e-10 490233.705051216 -602180.464147191;-0.000225 -8.95438662690012e-10 507061.746890568 -588080.560696902;-0.00015 -9.56687228501725e-10 523484.451327761 -573510.554644326;-7.5e-05 -1.01717103318078e-09 539488.690304143 -558482.093029373]  x2=[-0.000675 4.73912565734992e-09 369322.642211686 -697989.5746108;-0.0006 4.66666036101226e-09 388907.582416563 -687269.59463847;-0.000525 4.59046460778431e-09 408181.635850542 -676000.221867764;-0.00045 4.51059930738535e-09 427129.39513021 -664190.464862847;-0.000375 4.42712830291456e-09 445735.71370671 -651849.764162774;-0.0003 4.34011831981575e-09 463985.717973658 -638987.984734865;-0.000225 4.24963891253812e-09 481864.819156877 -625615.408088803;-0.00015 4.15576240893545e-09 499358.724976442 -611742.724057751;-7.5e-05 4.05856385244839e-09 516453.451071705 -597381.022253065]  x3=[-0.000675 1.55293323667891e-11 1409.06764658893 -5515.47701855251;-0.0006 1.73497033626054e-11 1564.42956176195 -5473.43717855389;-0.000525 1.91562052710129e-11 1718.54089587987 -5427.02195662112;-0.00045 2.09473940020266e-11 1871.27845470018 -5376.26845637245;-0.000375 2.27218377067809e-11 2022.52014215532 -5321.21724937943;-0.0003 2.44781179221282e-11 2172.14505795442 -5261.9123427346;-0.000225 2.62148307045364e-11 2320.03359422913 -5198.40114387295;-0.00015 2.79305877523796e-11 2466.06753114631 -5130.73442267509;-7.5e-05 2.9624017515726e-11 2610.13013141119 -5058.96627088262]  x4=[-0.000675 -2.91753763031922e-12 5928.29142347538 -10182.419728834;-0.0006 -5.37121402889565e-12 6213.78510946725 -10010.7531725412;-0.000525 -7.82059676115972e-12 6494.31159071671 -9831.08417333197;-0.00045 -1.02637278280321e-11 6769.64661864685 -9643.55635585521;-0.000375 -1.2698654227919e-11 7039.57009464911 -9448.31962697895;-0.0003 -1.5123429517912e-11 7303.86624602674 -9245.53005595701;-0.000225 -1.75361153697447e-11 7562.3237984802 -9035.34974966969;-0.00015 -1.99347831192623e-11 7814.73614499659 -8817.94672303798;-7.5e-05 -2.23175153081668e-11 8060.90151100814 -8593.49476471498]  x5=0.000667339049054976  V1=ones(3,3)  V2=ones(3,3)  I1=ones(3,3)  I2=ones(3,3)  nHarmo=1  Measurements=None  Decoupling=on  VsMag0=[634009.111289899 634008.470411727 634009.201310701]  VrMag0=[644768.423999943 644767.634896107 644768.519320875]  VsAngle0=[15.6289474446876 -104.371009723423 135.62901901781]  VrAngle0=[12.4643674245489 -107.535582309766 132.464453284623]  IsMag0=[4660.90997377981 4660.90842170561 4660.92192965338]  IrMag0=[9647.08196528286 9647.06470090305 9647.0719365125]  IsAngle0=[-1.08892209655233 -121.088741372843 118.911184788477]  IrAngle0=[14.7883279717862 -105.211681606019 134.788411982022]
      settings: AttributesFormatString=\n  LibrarySourceBlock=sps_lib/Power Grid Elements/Distributed Parameters Line
  LMO 330 Mvar : spsThreePhaseSeriesRLCLoadLib/Three-Phase Series RLC Load  LConnTagsString=A|B|C  Configuration=Y (grounded)  NominalVoltage=735e3  Vabc=[1e3 1e3 1e3]  Vabcp=[1e3 1e3 1e3]  NominalFrequency=60  UnbalancedPower=off  ActivePower=1100000  InductivePower=330e6  CapacitivePower=0  Pabc=[10e3 9e3 11e3]  QLabc=[100 90 110]  QCabc=[100 90 110]  Pabcp=[10e3 9e3 11e3]  QLabcp=[100 90 110]  QCabcp=[100 90 110]  Measurements=None  LoadType=constant Z
  LMO-ALB 3*218km : spsDistributedParametersLineLib/Distributed Parameters Line  Phases=3  Length=218  Frequency=60  Resistance="[0.01273  0.3864]/3"  Inductance="[0.9337e-3  4.1264e-3]/3"  Capacitance=[12.74e-9 7.751e-9]*3  x1=[-0.001275 5.17824676075131e-09 0 0;-0.0012 5.13745091383293e-09 0 0;-0.001125 5.09254826725967e-09 0 0;-0.00105 5.04357471552016e-09 0 0;-0.000975 4.99056940732235e-09 0 0;-0.0009 4.93357471429859e-09 0 0;-0.000825 4.87263619713445e-09 329282.961098438 -717747.524634889;-0.00075 4.80780256914815e-09 349442.471137451 -708151.592396784;-0.000675 4.73912565734992e-09 369322.642211686 -697989.5746108;-0.0006 4.66666036101226e-09 388907.582416563 -687269.59463847;-0.000525 4.59046460778431e-09 408181.635850542 -676000.221867764;-0.00045 4.51059930738535e-09 427129.39513021 -664190.464862847;-0.000375 4.42712830291456e-09 445735.71370671 -651849.764162774;-0.0003 4.34011831981575e-09 463985.717973658 -638987.984734865;-0.000225 4.24963891253812e-09 481864.819156877 -625615.408088803;-0.00015 4.15576240893545e-09 499358.724976442 -611742.724057751;-7.5e-05 4.05856385244839e-09 516453.451071705 -597381.022253065]  x2=[-0.001275 1.68686391265007e-08 0 0;-0.0012 1.68869409416196e-08 0 0;-0.001125 1.68917435945287e-08 0 0;-0.00105 1.68830432460606e-08 0 0;-0.000975 1.68608468511409e-08 0 0;-0.0009 1.6825172153228e-08 0 0;-0.000825 1.67760476701295e-08 208359.206060451 -779372.311348026;-0.00075 1.67135126712057e-08 230309.218727079 -773170.3359529;-0.000675 1.66376171459778e-08 252075.125728106 -766350.300021115;-0.0006 1.65484217641675e-08 273639.527730504 -758917.655385047;-0.000525 1.64459978271983e-08 294985.186481259 -750878.343587093;-0.00045 1.63304272111983e-08 316095.038587367 -742238.7911301;-0.000375 1.62018023015495e-08 336952.209156043 -733005.904340111;-0.0003 1.60602259190367e-08 357540.025284263 -723187.06384556;-0.000225 1.5905811237654e-08 377842.029386815 -712790.118677303;-0.00015 1.57386816941349e-08 397841.992352253 -701823.379994231;-7.5e-05 1.55589708892795e-08 417523.926516191 -690295.614439449]  x3=[-0.001275 2.66196099852489e-11 0 0;-0.0012 2.94305505383007e-11 0 0;-0.001125 3.22179647595546e-11 0 0;-0.00105 3.49796244327311e-11 0 0;-0.000975 3.77133219293423e-11 0 0;-0.0009 4.04168719734364e-11 0 0;-0.000825 4.30881133884738e-11 -103.698287435227 -3735.86307130135;-0.00075 4.57249108249386e-11 1.95817417063836 -3737.30097846037;-0.000675 4.83251564673047e-11 107.613070442033 -3735.75134439983;-0.0006 5.08867717189904e-11 213.181942471451 -3731.21540787349;-0.000525 5.34077088639577e-11 318.580400117851 -3723.69679483961;-0.00045 5.58859527036245e-11 423.72418946684 -3713.2015155624;-0.000375 5.83195221677838e-11 528.529260181966 -3699.73795980754;-0.0003 6.07064718982407e-11 632.911832693272 -3683.3168901355;-0.000225 6.30448938039024e-11 736.788465169399 -3663.95143329813;-0.00015 6.53329185860764e-11 840.076120219711 -3641.65706974531;-7.5e-05 6.756871723276e-11 942.692231273115 -3616.45162125016]  x4=[-0.001275 6.07374216158724e-11 0 0;-0.0012 5.83650853604763e-11 0 0;-0.001125 5.59460929488588e-11 0 0;-0.00105 5.3482378086542e-11 0 0;-0.000975 5.09759102294905e-11 0 0;-0.0009 4.84286930097592e-11 0 0;-0.000825 4.58427626338197e-11 3660.6608393673 -13572.4875623741;-0.00075 4.32201862548486e-11 4042.89932356741 -13463.5735253612;-0.000675 4.05630603202763e-11 4421.90597590669 -13343.8969136718;-0.0006 3.78735088959197e-11 4797.37782426627 -13213.553394958;-0.000525 3.51536819680358e-11 5169.01472219547 -13072.6471638344;-0.00045 3.2405753724656e-11 5536.51958884432 -12921.2908585863;-0.000375 2.96319208175734e-11 5899.59864644545 -12759.6054711282;-0.0003 2.68344006063727e-11 6257.96165515549 -12587.720250285;-0.000225 2.40154293859075e-11 6611.32214506842 -12405.7725984723;-0.00015 2.11772605986396e-11 6959.3976452152 -12213.9079618591;-7.5e-05 1.8322163033272e-11 7301.90990936676 -12012.2797141002]  x5=0.00123288061605072  V1=ones(3,3)  V2=ones(3,3)  I1=ones(3,3)  I2=ones(3,3)  nHarmo=1  Measurements=None  Decoupling=on  VsMag0=[644768.423999943 644767.634896107 644768.519320875]  VrMag0=[658703.501124853 658702.724611065 658703.398472819]  VsAngle0=[12.4643674245489 -107.535582309766 132.464453284623]  VrAngle0=[2.78756158795041 -117.212409726225 122.787634425017]  IsMag0=[3067.18219524945 3067.16950451033 3067.17450389731]  IrMag0=[11536.8651760446 11536.8607652588 11536.8706203315]  IsAngle0=[-13.7698967097865 -133.769925743268 106.230294079525]  IrAngle0=[2.91418185479763 -117.085774277233 122.914222759385]
      settings: AttributesFormatString=\n  LibrarySourceBlock=sps_lib/Power Grid Elements/Distributed Parameters Line
  LMO7 : spsThreePhaseVIMeasurementLib/Three-Phase V-I Measurement  VoltageMeasurement=no  SetLabelV=on  LabelV=Vabc_LMO7  Vpu=on  VpuLL=off  CurrentMeasurement=no  SetLabelI=off  LabelI=A1  Ipu=off  Pbase=100e6  Vbase=735e3  OutputType=Magnitude  PhasorSimulation=off  PSBequivalent=0
  LVD 990 Mvar : spsThreePhaseSeriesRLCLoadLib/Three-Phase Series RLC Load  LConnTagsString=A|B|C  Configuration=Y (grounded)  NominalVoltage=735e3  Vabc=[1e3 1e3 1e3]  Vabcp=[1e3 1e3 1e3]  NominalFrequency=60  UnbalancedPower=off  ActivePower=3300000  InductivePower=990e6  CapacitivePower=0  Pabc=[10e3 9e3 11e3]  QLabc=[100 90 110]  QCabc=[100 90 110]  Pabcp=[10e3 9e3 11e3]  QLabcp=[100 90 110]  QCabcp=[100 90 110]  Measurements=None  LoadType=constant Z
  LVD-MTL 3*260km : spsDistributedParametersLineLib/Distributed Parameters Line  Phases=3  Length=260  Frequency=60  Resistance="[0.01273  0.3864]/3"  Inductance="[0.9337e-3  4.1264e-3]/3"  Capacitance=[12.74e-9 7.751e-9]*3  x1=[-0.0015 5.824465354462e-08 -149994.752695009 -815900.545010832;-0.001425 5.84429069757938e-08 -126868.831368592 -819814.854171745;-0.00135 5.85944420413376e-08 -103641.493039537 -823073.815881822;-0.001275 5.86991376064386e-08 -80331.3052867147 -825674.824976934;-0.0012 5.87569099790639e-08 -56956.901917556 -827615.802250208;-0.001125 5.87677129768628e-08 -33536.9680724742 -828895.19611411;-0.00105 5.87315379640841e-08 -10090.2252882482 -829511.98384076;-0.000975 5.86484138584797e-08 13364.5834676878 -829465.672379487;-0.0009 5.85184071081876e-08 36808.7087800845 -828756.298750964;-0.000825 5.83416216386149e-08 60223.4097738746 -827384.430017616;-0.00075 5.8118198769361e-08 83589.9690953405 -825351.162830318;-0.000675 5.78483171012491e-08 106889.707874481 -822658.122551749;-0.0006 5.75321923735554e-08 130104.000656614 -819307.461957105;-0.000525 5.71700772915504e-08 153214.29029128 -815301.859513196;-0.00045 5.676226132449e-08 176202.102766545 -810644.51723733;-0.000375 5.63090704742186e-08 199049.06197684 -805339.15813766;-0.0003 5.58108670145677e-08 221736.904412544 -799390.023237078;-0.000225 5.52680492017603e-08 244247.493759549 -792801.868182998;-0.00015 5.46810509560505e-08 266562.835397155 -785579.959445767;-7.5e-05 5.40503415148546e-08 288665.090782692 -777730.070108732]  x2=[-0.0015 8.97002658537124e-08 -353353.509255483 -707507.476280055;-0.001425 8.98850941839073e-08 -333210.629182378 -717214.19053799;-0.00135 8.99980697450996e-08 -312801.385630599 -726347.574745754;-0.001275 9.00391022263543e-08 -292142.093437168 -734900.327815756;-0.0012 9.00081588269338e-08 -271249.267324168 -742865.612808055;-0.001125 8.9905264282518e-08 -250139.608697122 -750237.062395701;-0.00105 8.97305008454314e-08 -228829.992294147 -757008.783954679;-0.000975 8.94840082188917e-08 -207337.452696549 -763175.364274386;-0.0009 8.9165983445333e-08 -185679.170711635 -768731.873884868;-0.000825 8.87766807488935e-08 -163872.45963864 -773673.870997357;-0.00075 8.8316411332192e-08 -141934.751428743 -777997.405054979;-0.000675 8.7785543127558e-08 -119883.582750228 -781699.019890759;-0.0006 8.71845005029116e-08 -97736.5809699434 -784775.756490435;-0.000525 8.65137639225309e-08 -75511.450062251 -787225.155357843;-0.00045 8.57738695629754e-08 -53225.9564567427 -789045.258481008;-0.000375 8.49654088844755e-08 -30897.9148360274 -790234.61089734;-0.0003 8.40890281581278e-08 -8545.1738949461 -790792.261856716;-0.000225 8.31454279492756e-08 13814.3979274013 -790717.765581491;-0.00015 8.21353625574886e-08 36162.9267314129 -790011.181622847;-7.5e-05 8.10596394135862e-08 58482.5474451067 -788673.074813191]  x3=[-0.0015 2.59057047829938e-10 176.513539923912 -1804.55713842473;-0.001425 2.67619956269538e-10 227.459268205972 -1798.84517601327;-0.00135 2.75968933410819e-10 278.22316902927 -1791.69524429136;-0.001275 2.84097305209198e-10 328.764662508205 -1783.11305880501;-0.0012 2.91998573968627e-10 379.043346546198 -1773.105480022;-0.001125 2.99666423535753e-10 429.01902913252 -1761.68050784769;-0.00105 3.07094724348955e-10 478.651760471164 -1748.84727523001;-0.000975 3.14277538338219e-10 527.901864916106 -1734.61604085878;-0.0009 3.21209123671943e-10 576.729972687402 -1718.998180965;-0.000825 3.27883939346868e-10 625.097051342797 -1702.00618022692;-0.00075 3.34296649617472e-10 672.964436979654 -1683.65362178992;-0.000675 3.40442128261282e-10 720.293865142291 -1663.95517640844;-0.0006 3.46315462676699e-10 767.047501409999 -1642.9265907183;-0.000525 3.51911957810056e-10 813.1879716413 -1620.58467464916;-0.00045 3.57227139908774e-10 858.678391850264 -1596.94728798688;-0.000375 3.62256760097607e-10 903.482397691003 -1572.03332609669;-0.0003 3.66996797775133e-10 947.564173526772 -1545.86270481855;-0.000225 3.71443463827756e-10 990.888481060442 -1518.45634454666;-0.00015 3.75593203658671e-10 1033.42068750345 -1489.8361535061;-7.5e-05 3.7944270002935e-10 1075.12679326074 -1460.02501023969]  x4=[-0.0015 2.73276882598602e-10 -8566.49009753155 -13975.6180438616;-0.001425 2.70534584511781e-10 -8167.96786665192 -14212.2119177621;-0.00135 2.67576025217419e-10 -7762.9162872338 -14437.4447669097;-0.001275 2.64403569742549e-10 -7351.65915131226 -14651.1365436109;-0.0012 2.61019754099538e-10 -6934.52521154932 -14853.1164259291;-0.001125 2.57427283258835e-10 -6511.84791843406 -15043.2229542367;-0.00105 2.53629028986664e-10 -6083.96515372742 -15221.3041602837;-0.000975 2.49628027549376e-10 -5651.21896036468 -15387.2176886787;-0.0009 2.45427477286302e-10 -5213.95526903157 -15540.8309106858;-0.000825 2.41030736053051e-10 -4772.52362163259 -15682.0210302455;-0.00075 2.36441318537294e-10 -4327.27689187254 -15810.6751821366;-0.000675 2.31662893449171e-10 -3878.57100317468 -15926.6905221985;-0.0006 2.26699280588586e-10 -3426.764644161 -16029.9743095435;-0.000525 2.21554447791714e-10 -2972.21898192205 -16120.4439806923;-0.00045 2.16232507759174e-10 -2515.29737330542 -16198.0272155741;-0.000375 2.107377147684e-10 -2056.36507445391 -16262.6619953378;-0.0003 2.05074461272835e-10 -1595.78894882532 -16314.2966519295;-0.000225 1.99247274390673e-10 -1133.93717392743 -16352.8899093947;-0.00015 1.93260812285949e-10 -671.178947002525 -16378.410916874;-7.5e-05 1.87119860444872e-10 -207.884189896768 -16390.8392732645]  x5=0.00147040807418893  V1=ones(3,3)  V2=ones(3,3)  I1=ones(3,3)  I2=ones(3,3)  nHarmo=1  Measurements=None  Decoupling=on  VsMag0=[677344.070714008 677343.614711332 677343.797959469]  VrMag0=[645717.103800436 645717.117585008 645716.873803144]  VsAngle0=[-8.01690098277627 -128.01690535406 111.983130236585]  VrAngle0=[-24.139092789334 -144.139117060794 95.8608940156766]  IsMag0=[1489.54148608122 1489.52649322658 1489.52592422232]  IrMag0=[13466.1974570842 13466.198803439 13466.2083731084]  IsAngle0=[7.98693859743065 -112.013419640751 127.987258926355]  IrAngle0=[-29.1066680799871 -149.106617756849 90.8933521206054]
      settings: AttributesFormatString=\n  LibrarySourceBlock=sps_lib/Power Grid Elements/Distributed Parameters Line
  LVD7 : spsThreePhaseVIMeasurementLib/Three-Phase V-I Measurement  VoltageMeasurement=no  SetLabelV=on  LabelV=Vabc_LVD7  Vpu=on  VpuLL=off  CurrentMeasurement=no  SetLabelI=off  LabelI=A1  Ipu=off  Pbase=100e6  Vbase=735e3  OutputType=Magnitude  PhasorSimulation=off  PSBequivalent=0
  Load Flow Bus1 : spsLoadFlowBusLib/Load Flow Bus  LConnTagsString=a  Phases=single  Connectors=on one side  ID=LG31_13.8  Vbase=13.8e3  Vref=1  Vangle=0  VLF=1  VLFb=1  VLFc=1  angleLF=-0.0351  angleLFb=0  angleLFc=0
      settings: AttributesFormatString=%<ID>\n%<Vbase>V\n%<VLF>pu\n%<angleLF>deg.
  Load Flow Bus10 : spsLoadFlowBusLib/Load Flow Bus  LConnTagsString=a  Phases=single  Connectors=on one side  ID=LVD7  Vbase=735e3  Vref=1  Vangle=0  VLF=1.05  VLFb=1  VLFc=1  angleLF=-12.02  angleLFb=0  angleLFc=0
      settings: AttributesFormatString=%<ID>\n%<Vbase>V\n%<VLF>pu\n%<angleLF>deg.
  Load Flow Bus11 : spsLoadFlowBusLib/Load Flow Bus  LConnTagsString=a  Phases=single  Connectors=on one side  ID=CHM7  Vbase=735e3  Vref=1  Vangle=0  VLF=1.047  VLFb=1  VLFc=1  angleLF=-4.064  angleLFb=0  angleLFc=0
      settings: AttributesFormatString=%<ID>\n%<Vbase>V\n%<VLF>pu\n%<angleLF>deg.
  Load Flow Bus12 : spsLoadFlowBusLib/Load Flow Bus  LConnTagsString=a  Phases=single  Connectors=on one side  ID=LG47  Vbase=735e3  Vref=1  Vangle=0  VLF=1.004  VLFb=1  VLFc=1  angleLF=20.71  angleLFb=0  angleLFc=0
      settings: AttributesFormatString=%<ID>\n%<Vbase>V\n%<VLF>pu\n%<angleLF>deg.
  Load Flow Bus2 : spsLoadFlowBusLib/Load Flow Bus  LConnTagsString=a  Phases=single  Connectors=on one side  ID=LG3_13.8  Vbase=13.8e3  Vref=1  Vangle=0  VLF=1  VLFb=1  VLFc=1  angleLF=-0.6025  angleLFb=0  angleLFc=0
      settings: AttributesFormatString=%<ID>\n%<Vbase>V\n%<VLF>pu\n%<angleLF>deg.
  Load Flow Bus3 : spsLoadFlowBusLib/Load Flow Bus  LConnTagsString=a  Phases=single  Connectors=on one side  ID=LG4_13.8  Vbase=13.8e3  Vref=1  Vangle=0  VLF=1  VLFb=1  VLFc=1  angleLF=-3.293  angleLFb=0  angleLFc=0
      settings: AttributesFormatString=%<ID>\n%<Vbase>V\n%<VLF>pu\n%<angleLF>deg.
  Load Flow Bus4 : spsLoadFlowBusLib/Load Flow Bus  LConnTagsString=a  Phases=single  Connectors=on one side  ID=LG2_13.8  Vbase=13.8e3  Vref=1  Vangle=0  VLF=1  VLFb=1  VLFc=1  angleLF=0  angleLFb=0  angleLFc=0
      settings: AttributesFormatString=%<ID>\n%<Vbase>V\n%<VLF>pu\n%<angleLF>deg.
  Load Flow Bus5 : spsLoadFlowBusLib/Load Flow Bus  LConnTagsString=a  Phases=single  Connectors=on one side  ID=LG27  Vbase=735e3  Vref=1  Vangle=0  VLF=1  VLFb=1  VLFc=1  angleLF=23.57  angleLFb=0  angleLFc=0
      settings: AttributesFormatString=%<ID>\n%<Vbase>V\n%<VLF>pu\n%<angleLF>deg.
  Load Flow Bus6 : spsLoadFlowBusLib/Load Flow Bus  LConnTagsString=a  Phases=single  Connectors=on one side  ID=LG37  Vbase=735e3  Vref=1  Vangle=0  VLF=0.994  VLFb=1  VLFc=1  angleLF=24.1  angleLFb=0  angleLFc=0
      settings: AttributesFormatString=%<ID>\n%<Vbase>V\n%<VLF>pu\n%<angleLF>deg.
  Load Flow Bus7 : spsLoadFlowBusLib/Load Flow Bus  LConnTagsString=a  Phases=single  Connectors=on one side  ID=LMO7  Vbase=735e3  Vref=1  Vangle=0  VLF=1.016  VLFb=1  VLFc=1  angleLF=17.31  angleLFb=0  angleLFc=0
      settings: AttributesFormatString=%<ID>\n%<Vbase>V\n%<VLF>pu\n%<angleLF>deg.
  Load Flow Bus8 : spsLoadFlowBusLib/Load Flow Bus  LConnTagsString=a  Phases=single  Connectors=on one side  ID=NEM_ALB7  Vbase=735e3  Vref=1  Vangle=0  VLF=1.028  VLFb=1  VLFc=1  angleLF=8.928  angleLFb=0  angleLFc=0
      settings: AttributesFormatString=%<ID>\n%<Vbase>V\n%<VLF>pu\n%<angleLF>deg.
  Load Flow Bus9 : spsLoadFlowBusLib/Load Flow Bus  LConnTagsString=a  Phases=single  Connectors=on one side  ID=ABI_CHB7  Vbase=735e3  Vref=1  Vangle=0  VLF=1.046  VLFb=1  VLFc=1  angleLF=0.1334  angleLFb=0  angleLFc=0
      settings: AttributesFormatString=%<ID>\n%<Vbase>V\n%<VLF>pu\n%<angleLF>deg.
  NEM-ABI 6*236 : spsDistributedParametersLineLib/Distributed Parameters Line  Phases=3  Length=236  Frequency=60  Resistance="[0.01273  0.3864]/6"  Inductance="[0.9337e-3  4.1264e-3]/6"  Capacitance=[12.74e-9 7.751e-9]*6  x1=[-0.00135 1.6248252489232e-08 0 0;-0.001275 1.62898333778589e-08 0 0;-0.0012 1.63183924229264e-08 0 0;-0.001125 1.63339067947707e-08 0 0;-0.00105 1.63363640914405e-08 0 0;-0.000975 1.63257623486103e-08 0 0;-0.0009 1.63021100411511e-08 0 0;-0.000825 1.62654260763557e-08 235173.13625179 -772031.41700735;-0.00075 1.62157397788243e-08 256904.899781766 -765074.329412325;-0.000675 1.61530908670228e-08 278431.297465632 -757505.653104398;-0.0006 1.60775294215327e-08 299735.121430446 -749331.438367604;-0.000525 1.59891158450176e-08 320799.34172529 -740558.219544135;-0.00045 1.58879208139376e-08 341607.119934753 -731193.009810882;-0.000375 1.57740252220523e-08 362141.822639305 -721243.295573215;-0.0003 1.56475201157551e-08 382387.034711794 -710717.03048046;-0.000225 1.55085066212926e-08 402326.572439453 -699622.629067873;-0.00015 1.5357095863925e-08 421944.496460906 -687968.960030195;-7.5e-05 1.51934088790953e-08 441225.124507856 -675765.339132147]  x2=[-0.00135 2.9400630950868e-08 0 0;-0.001275 2.94493865273734e-08 0 0;-0.0012 2.94746007148796e-08 0 0;-0.001125 2.94762533575507e-08 0 0;-0.00105 2.94543431342897e-08 0 0;-0.000975 2.94088875597937e-08 0 0;-0.0009 2.93399229705534e-08 0 0;-0.000825 2.92475044958063e-08 81706.5138318076 -820341.457427507;-0.00075 2.91317060134672e-08 104865.377019223 -817703.667465364;-0.000675 2.89926200910709e-08 127940.412428743 -814412.217702735;-0.0006 2.88303579117757e-08 150913.174230121 -810469.739274199;-0.000525 2.86450491854852e-08 173765.298349069 -805879.38373669;-0.00045 2.84368420451597e-08 196478.517147215 -800644.82055019;-0.000375 2.82059029284016e-08 219034.674024975 -794770.234144418;-0.0003 2.79524164444074e-08 241415.737935663 -788260.320573864;-0.000225 2.76765852263937e-08 263603.817799229 -781120.283763831;-0.00015 2.73786297696161e-08 285581.176804121 -773355.831350497;-7.5e-05 2.70587882551077e-08 307330.246585814 -764973.170118324]  x3=[-0.00135 1.58063340302713e-10 0 0;-0.001275 1.64813497783715e-10 0 0;-0.0012 1.71431905876321e-10 0 0;-0.001125 1.77913273926365e-10 0 0;-0.00105 1.84252420827396e-10 0 0;-0.000975 1.90444279162375e-10 0 0;-0.0009 1.96483899254487e-10 0 0;-0.000825 2.02366453123839e-10 -1379.76964294105 -6710.39772290172;-0.00075 2.08087238346874e-10 -1189.51028635693 -6746.72121821299;-0.000675 2.13641681815416e-10 -998.300053450018 -6777.65148781071;-0.0006 2.19025343392343e-10 -806.291794754879 -6803.16380651062;-0.000525 2.24233919460962e-10 -613.63899873569 -6823.23778015551;-0.00045 2.29263246365257e-10 -420.495669089904 -6837.85736191797;-0.000375 2.34109303738254e-10 -227.016201640046 -6847.01086512805;-0.0003 2.38768217715835e-10 -33.3552609120621 -6850.69097261532;-0.000225 2.4323626403345e-10 160.332343501142 -6848.89474255817;-0.00015 2.47509871003236e-10 353.891780692119 -6841.62361083543;-7.5e-05 2.5158562236917e-10 547.168322208337 -6828.88338987853]  x4=[-0.00135 1.75424368200249e-10 0 0;-0.001275 1.71621449420394e-10 0 0;-0.0012 1.67681339079769e-10 0 0;-0.001125 1.63607186842293e-10 0 0;-0.00105 1.5940224952293e-10 0 0;-0.000975 1.55069888484235e-10 0 0;-0.0009 1.50613566949334e-10 0 0;-0.000825 1.46036847233478e-10 2916.74328192147 -29367.0114378027;-0.00075 1.41343387896383e-10 3745.79818277931 -29272.8158501774;-0.000675 1.3653694081763e-10 4571.85874988247 -29155.2200214506;-0.0006 1.31621348197472e-10 5394.26464305276 -29014.3179559284;-0.000525 1.2660053948544e-10 6212.35844360241 -28850.2222885662;-0.00045 1.21478528239196e-10 7025.48617986451 -28663.0641949298;-0.000375 1.16259408916161e-10 7832.99784996797 -28452.9932863355;-0.0003 1.10947353600468e-10 8634.24794143906 -28220.1774902535;-0.000225 1.05546608667858e-10 9428.59594721418 -27964.802916069;-0.00015 1.00061491391196e-10 10215.4068776515 -27687.0737063092;-7.5e-05 9.44963864893075e-11 10994.0517681317 -27387.2118734551]  x5=0.00133467809810995  V1=ones(3,3)  V2=ones(3,3)  I1=ones(3,3)  I2=ones(3,3)  nHarmo=1  Measurements=None  Decoupling=on  VsMag0=[658958.583852861 658957.792322726 658958.516680741]  VrMag0=[673120.404843161 673119.992372414 673120.175209654]  VsAngle0=[4.76158286037793 -115.238384148893 124.76165895798]  VrAngle0=[-6.49205363089456 -126.492055930659 113.50797562484]  IsMag0=[5624.79821722864 5624.77239180534 5624.75565924819]  IrMag0=[24230.0809184618 24230.0884931979 24230.1137544068]  IsAngle0=[-23.7987124057266 -143.799061097514 96.2013410715065]  IrAngle0=[-6.50799783402815 -126.50791851781 113.492026312176]
      settings: AttributesFormatString=\n  LibrarySourceBlock=sps_lib/Power Grid Elements/Distributed Parameters Line
  NEM-ALB 1980 Mvar : spsThreePhaseSeriesRLCLoadLib/Three-Phase Series RLC Load  LConnTagsString=A|B|C  Configuration=Y (grounded)  NominalVoltage=735e3  Vabc=[1e3 1e3 1e3]  Vabcp=[1e3 1e3 1e3]  NominalFrequency=60  UnbalancedPower=off  ActivePower=6600000  InductivePower=1980e6  CapacitivePower=0  Pabc=[10e3 9e3 11e3]  QLabc=[100 90 110]  QCabc=[100 90 110]  Pabcp=[10e3 9e3 11e3]  QLabcp=[100 90 110]  QCabcp=[100 90 110]  Measurements=None  LoadType=constant Z
  NEM-ALB7 : spsThreePhaseVIMeasurementLib/Three-Phase V-I Measurement  VoltageMeasurement=no  SetLabelV=on  LabelV=Vabc_NEM7  Vpu=on  VpuLL=off  CurrentMeasurement=no  SetLabelI=off  LabelI=A1  Ipu=off  Pbase=100e6  Vbase=735e3  OutputType=Magnitude  PhasorSimulation=off  PSBequivalent=0
  Regulators1 : Subsystem
  Regulators2 : Subsystem
  Regulators3 : Subsystem
  Regulators4 : Subsystem
  MTLa : PMIOPort  Side=Right
  MTLb : PMIOPort  Port=2  Side=Right
  MTLc : PMIOPort  Port=3  Side=Right
  CHM7a : PMIOPort  Port=4  Side=Right
  CHM7b : PMIOPort  Port=5  Side=Right
  CHM7c : PMIOPort  Port=6  Side=Right
  wires:
  Regulators2/1(Pm) -> LG3_2200 MVA/1
  Regulators4/2(Vf) -> LG4-2700 MVA/2
  Regulators4/1(Pm) -> LG4-2700 MVA/1
  Regulators3/2(Vf) -> LG31-200 MVA/2
  Regulators3/1(Pm) -> LG31-200 MVA/1
  Regulators2/2(Vf) -> LG3_2200 MVA/2
  LG3_2200 MVA/1 -> Regulators2/1(m)
  Regulators1/1(Pm) -> LG2_5500 MVA/1
  Regulators1/2(Vf) -> LG2_5500 MVA/2
  LG2_5500 MVA/1 -> Regulators1/1(m)
  LG31-200 MVA/1 -> Regulators3/1(m)
  LG4-2700 MVA/1 -> Regulators4/1(m)
  connections:
  LG2-NENI 3*279km/RConn1 -- "Cs NEM "/LConn1
  LG2-NENI 3*279km/RConn2 -- "Cs NEM "/LConn2
  LG2-NENI 3*279km/RConn3 -- "Cs NEM "/LConn3
  CHB-CHM 3*195km/RConn1 -- "Cs  CHMN "/LConn1
  CHB-CHM 3*195km/RConn2 -- "Cs  CHMN "/LConn2
  CHB-CHM 3*195km/RConn3 -- "Cs  CHMN "/LConn3
  Load Flow Bus2/LConn1 -- 2200 MVA 13.8 kV/735 kV/LConn1 -- LG3_2200 MVA/RConn1 -- 110 MW/LConn1
  2200 MVA 13.8 kV/735 kV/LConn2 -- LG3_2200 MVA/RConn2 -- 110 MW/LConn2
  2200 MVA 13.8 kV/735 kV/LConn3 -- LG3_2200 MVA/RConn3 -- 110 MW/LConn3
  Load Flow Bus1/LConn1 -- 200 MVA 13.8 kV/735 kV/LConn1 -- LG31-200 MVA/RConn1 -- 10 MW/LConn1
  200 MVA 13.8 kV/735 kV/LConn2 -- LG31-200 MVA/RConn2 -- 10 MW/LConn2
  200 MVA 13.8 kV/735 kV/LConn3 -- LG31-200 MVA/RConn3 -- 10 MW/LConn3
  Load Flow Bus6/LConn1 -- 2200 MVA 13.8 kV/735 kV/RConn1 -- 200 MVA 13.8 kV/735 kV/RConn1 -- LG3-LMO 104km/LConn1 -- LG3 660 Mvar/LConn1 -- LG2-LG3 155km/RConn1
  2200 MVA 13.8 kV/735 kV/RConn2 -- LG3 660 Mvar/LConn2 -- LG2-LG3 155km/RConn2 -- 200 MVA 13.8 kV/735 kV/RConn2 -- LG3-LMO 104km/LConn2
  LG3-LMO 104km/RConn1 -- LMO7/RConn1 -- LG4-LMO 3*118km/RConn1 -- LMO 330 Mvar/LConn1
  LG3-LMO 104km/RConn2 -- LMO7/RConn2 -- LG4-LMO 3*118km/RConn2 -- LMO 330 Mvar/LConn2
  LG3-LMO 104km/RConn3 -- LMO7/RConn3 -- LG4-LMO 3*118km/RConn3 -- LMO 330 Mvar/LConn3
  LG4-LMO 3*118km/LConn1 -- LG4 660 Mvar/LConn1 -- 2700 MVA 13.8 kV/735 kV/RConn1 -- Load Flow Bus12/LConn1
  LG4-LMO 3*118km/LConn2 -- 2700 MVA 13.8 kV/735 kV/RConn2 -- LG4 660 Mvar/LConn2
  LG4 660 Mvar/LConn3 -- 2700 MVA 13.8 kV/735 kV/RConn3 -- LG4-LMO 3*118km/LConn3
  Load Flow Bus3/LConn1 -- LG4-2700 MVA/RConn1 -- 2700 MVA 13.8 kV/735 kV/LConn1 -- 135 MW/LConn1
  LG4-2700 MVA/RConn2 -- 2700 MVA 13.8 kV/735 kV/LConn2 -- 135 MW/LConn2
  LG4-2700 MVA/RConn3 -- 2700 MVA 13.8 kV/735 kV/LConn3 -- 135 MW/LConn3
  Load Flow Bus4/LConn1 -- 5500 MVA 13.8 kV/735 kV/LConn1 -- LG2_5500 MVA/RConn1 -- 275 MW/LConn1
  5500 MVA 13.8 kV/735 kV/LConn2 -- LG2_5500 MVA/RConn2 -- 275 MW/LConn2
  LG2_5500 MVA/RConn3 -- 5500 MVA 13.8 kV/735 kV/LConn3 -- 275 MW/LConn3
  5500 MVA 13.8 kV/735 kV/RConn1 -- LG2-NENI 3*279km/LConn1 -- LG2-LG3 155km/LConn1 -- LG2 660 Mvar/LConn1 -- Load Flow Bus5/LConn1
  LG2-LG3 155km/LConn2 -- 5500 MVA 13.8 kV/735 kV/RConn2 -- LG2-NENI 3*279km/LConn2 -- LG2 660 Mvar/LConn2
  LG2-LG3 155km/LConn3 -- 5500 MVA 13.8 kV/735 kV/RConn3 -- LG2-NENI 3*279km/LConn3 -- LG2 660 Mvar/LConn3
  "Cs NEM "/RConn1 -- NEM-ALB7/LConn1 -- Cs ALB/RConn1
  "Cs NEM "/RConn2 -- NEM-ALB7/LConn2 -- Cs ALB/RConn2
  "Cs NEM "/RConn3 -- NEM-ALB7/LConn3 -- Cs ALB/RConn3
  LMO7/LConn1 -- LMO-ALB 3*218km/LConn1
  LMO7/LConn2 -- LMO-ALB 3*218km/LConn2
  Load Flow Bus7/LConn1 -- LMO7/LConn3 -- LMO-ALB 3*218km/LConn3
  Cs ALB/LConn1 -- LMO-ALB 3*218km/RConn1
  Cs ALB/LConn2 -- LMO-ALB 3*218km/RConn2
  Cs ALB/LConn3 -- LMO-ALB 3*218km/RConn3
  200 MVA 13.8 kV/735 kV/RConn3 -- LG3-LMO 104km/LConn3 -- LG3 660 Mvar/LConn3 -- LG2-LG3 155km/RConn3 -- 2200 MVA 13.8 kV/735 kV/RConn3
  Load Flow Bus8/LConn1 -- NEM-ABI 6*236/LConn1 -- NEM-ALB7/RConn1 -- NEM-ALB 1980 Mvar/LConn1
  NEM-ALB 1980 Mvar/LConn2 -- NEM-ALB7/RConn2 -- NEM-ABI 6*236/LConn2
  NEM-ALB 1980 Mvar/LConn3 -- NEM-ALB7/RConn3 -- NEM-ABI 6*236/LConn3
  NEM-ABI 6*236/RConn1 -- "Cs ABI+CHB "/LConn1
  NEM-ABI 6*236/RConn2 -- "Cs ABI+CHB "/LConn2
  NEM-ABI 6*236/RConn3 -- "Cs ABI+CHB "/LConn3
  "Cs ABI+CHB "/RConn1 -- ABI-CHB7/LConn1
  "Cs ABI+CHB "/RConn2 -- ABI-CHB7/LConn2
  "Cs ABI+CHB "/RConn3 -- ABI-CHB7/LConn3
  Load Flow Bus9/LConn1 -- ABI+CHB 1320 Mvar/LConn1 -- CHB-CHM 3*195km/LConn1 -- ABI-CHB 3*271km/LConn1 -- ABI-CHB7/RConn1
  ABI-CHB 3*271km/LConn2 -- ABI-CHB7/RConn2 -- ABI+CHB 1320 Mvar/LConn2 -- CHB-CHM 3*195km/LConn2
  ABI-CHB 3*271km/LConn3 -- ABI-CHB7/RConn3 -- ABI+CHB 1320 Mvar/LConn3 -- CHB-CHM 3*195km/LConn3
  ABI-CHB 3*271km/RConn1 -- "Cs LVDN "/LConn1
  ABI-CHB 3*271km/RConn2 -- "Cs LVDN "/LConn2
  ABI-CHB 3*271km/RConn3 -- "Cs LVDN "/LConn3
  "Cs LVDN "/RConn1 -- LVD7/LConn1
  "Cs LVDN "/RConn2 -- LVD7/LConn2
  "Cs LVDN "/RConn3 -- LVD7/LConn3
  "Cs LVDS "/LConn1 -- LVD 990 Mvar/LConn1 -- Load Flow Bus10/LConn1 -- LVD7/RConn1
  "Cs LVDS "/LConn2 -- LVD7/RConn2 -- LVD 990 Mvar/LConn2
  "Cs LVDS "/LConn3 -- LVD7/RConn3 -- LVD 990 Mvar/LConn3
  "Cs LVDS "/RConn1 -- LVD-MTL 3*260km/LConn1
  "Cs LVDS "/RConn2 -- LVD-MTL 3*260km/LConn2
  "Cs LVDS "/RConn3 -- LVD-MTL 3*260km/LConn3
  MTLa/RConn1 -- LVD-MTL 3*260km/RConn1
  MTLb/RConn1 -- LVD-MTL 3*260km/RConn2
  MTLc/RConn1 -- LVD-MTL 3*260km/RConn3
  "Cs  CHMN "/RConn1 -- CHM7/LConn1
  "Cs  CHMN "/RConn2 -- CHM7/LConn2
  "Cs  CHMN "/RConn3 -- CHM7/LConn3
  CHM 1320Mvar/LConn2 -- CHM7/RConn2 -- CHM7b/RConn1
  Load Flow Bus11/LConn1 -- CHM 1320Mvar/LConn3 -- CHM7c/RConn1 -- CHM7/RConn3
  CHM7a/RConn1 -- CHM 1320Mvar/LConn1 -- CHM7/RConn1
